simulink model "create_rc_params_Preq"  (Simulink 3.00)
settings: Solver=ode1  StartTime=starttime  StopTime=endtime  FixedStep=0.5  RelTol=1e-3
values from neighbouring files (symbols this model uses):
  cb = energy/(0.5*(Vmax^2-Vmin^2))    [process_HPPC.m]
  cc = tau/(re+rt)    [process_HPPC.m]
  ess_max_volts = template_max_volts    [ESS_RC_template.m]    (also in ESS_template.m)
  ess_min_volts = template_min_volts    [ESS_RC_template.m]    (also in ESS_template.m)
  ess_mod_airflow = max(ess_mod_airflow,0.001)    [ESS_RC_template.m]    (also in ESS_template.m)
  ess_mod_cp = template_mod_cp    [ESS_RC_template.m]    (also in ESS_template.m)
  ess_module_mass = template_module_mass    [ESS_RC_template.m]    (also in ESS_template.m)
  ess_module_num = template_module_num    [ESS_RC_template.m]    (also in ESS_template.m)
  ess_set_tmp = template_set_tmp    [ESS_RC_template.m]    (also in ESS_template.m)
  ess_soc = template_soc    [ESS_RC_template.m]    (also in ESS_template.m; make_ADV_RC_bat_file.m = binf.VOC.ess_soc/100; make_ADV_bat_file.m = binf.VOC.ess_soc; process_HPPC.m = [0:.2:min_soc-.2 min_soc:.05:max_soc max_soc+.2:.2:1])
  ess_th_calc = 1    [ESS_RC_template.m]    (also in ESS_template.m)
  ess_th_res_off = ((1/4)+(ess_mod_case_thk/ess_mod_case_th_cond))/ess_mod_sarea    [ESS_RC_template.m]    (also in ESS_template.m)
  ess_th_res_on = min(ess_th_res_on,ess_th_res_off)    [ESS_RC_template.m]    (also in ESS_template.m)
  ess_tmp = template_tmp    [ESS_RC_template.m]    (also in ESS_template.m; process_HPPC.m = [1 1.01]*Temperature)
  ess_voc = template_voc    [ESS_RC_template.m]    (also in ESS_template.m = template_voc*templatenum_cells_per_mod; process_HPPC.m = [ess_voc_data;ess_voc_data]; process_data.m = binf.VOC.ess_voc)
  mc_min_volts = 0    [validate_rc.m]
  rc = Rbulk/3.732*factor    [process_HPPC.m]
  re = Rbulk/(1.244)    [process_HPPC.m]
  rt = Rbulk/1.368*factor    [process_HPPC.m]
undefined symbols (not defined in the file or in its folder): air_cp, amb_tmp, cyc_mph, ess_init_soc, ess_mod_init_tmp, power_data, time_data
settings Model: LastModifiedBy=vjohnson

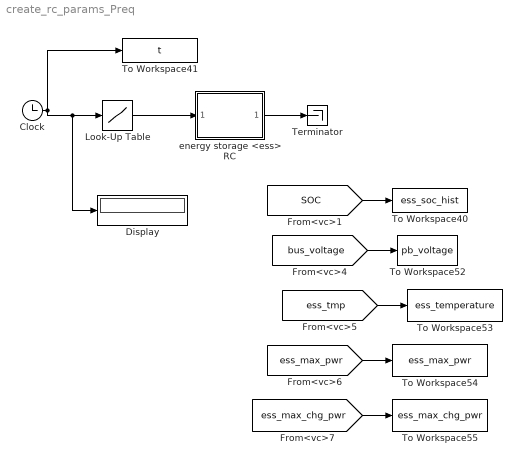
== system create_rc_params_Preq ==
  Clock : Clock
      settings: DisplayTime=off  Decimation=10
  Display : Display
      settings: Format=short
  Look-Up Table : Lookup  InputValues=time_data  OutputValues=power_data
  Terminator : Terminator
  To Workspace40 : ToWorkspace  VariableName=ess_soc_hist  SampleTime=-1  SaveFormat=Matrix
  To Workspace41 : ToWorkspace  VariableName=t  SampleTime=-1  SaveFormat=Matrix
  To Workspace52 : ToWorkspace  VariableName=pb_voltage  SampleTime=-1  SaveFormat=Matrix
  To Workspace53 : ToWorkspace  VariableName=ess_temperature  SampleTime=-1  SaveFormat=Matrix
  To Workspace54 : ToWorkspace  VariableName=ess_max_pwr  SampleTime=-1  SaveFormat=Matrix
  To Workspace55 : ToWorkspace  VariableName=ess_max_chg_pwr  SampleTime=-1  SaveFormat=Matrix
  energy storage <ess> RC : Subsystem
      mask Display: image(imread('bdi_ess.jpg'))
  wires:
  Look-Up Table/1 -> energy storage <ess> RC/1(power req'd into bus (W))
  energy storage <ess> RC/1(power available to bus (W)) -> Terminator/1
  [bus_voltage] -> To Workspace52/1
  [SOC] -> To Workspace40/1
  [ess_tmp] -> To Workspace53/1
  [ess_max_pwr] -> To Workspace54/1
  [ess_max_chg_pwr] -> To Workspace55/1
  Clock/1 -> To Workspace41/1, Look-Up Table/1, Display/1

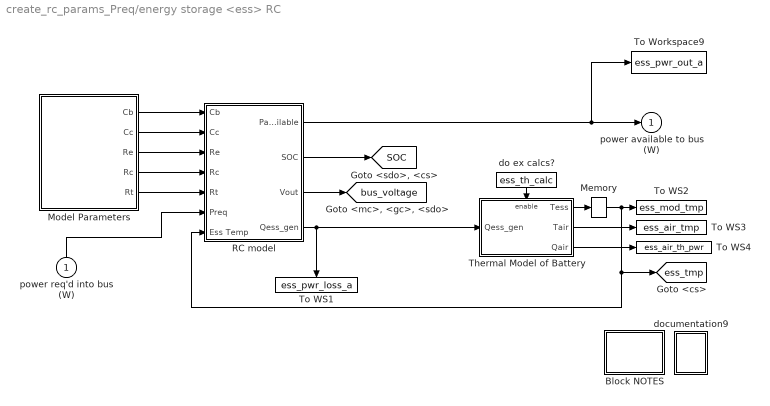
== system create_rc_params_Preq/energy storage <ess> RC ==
  power req'd into bus (W) : Inport  Orientation=up  Port=1  PortWidth=-1  SampleTime=-1  DataType=auto
      settings: SignalType=auto
  Block NOTES : Subsystem
      mask Display: disp('Block\nNOTES')
  Memory : Memory  X0=ess_mod_init_tmp  InheritSampleTime=off
  Model Parameters : Subsystem
  RC model : Subsystem
  Thermal Model of Battery : Subsystem
  To WS1 : ToWorkspace  VariableName=ess_pwr_loss_a  SampleTime=0  SaveFormat=Matrix
      settings: Orientation=down
  To WS2 : ToWorkspace  VariableName=ess_mod_tmp  SampleTime=0  SaveFormat=Matrix
  To WS3 : ToWorkspace  VariableName=ess_air_tmp  SampleTime=0  SaveFormat=Matrix
  To WS4 : ToWorkspace  VariableName=ess_air_th_pwr  SampleTime=0  SaveFormat=Matrix
  To Workspace9 : ToWorkspace  VariableName=ess_pwr_out_a  SampleTime=-1  SaveFormat=Matrix
  do ex calcs? : Constant  Orientation=down  Value=ess_th_calc
  documentation9 : Subsystem
      settings: OpenFcn=web(['file:\\\' which('energy_storage.htm')]);
      mask Display: image(imread('doc_man.jpg'))
  power available to bus (W) : Outport  Port=1  InitialOutput=0
  tag scope: SOC=global, bus_voltage=global, ess_tmp=global
  wires:
  Model Parameters/1(Cb) -> RC model/1(Cb)
  Model Parameters/2(Cc) -> RC model/2(Cc)
  Model Parameters/3(Re) -> RC model/3(Re)
  Model Parameters/4(Rc) -> RC model/4(Rc)
  Model Parameters/5(Rt) -> RC model/5(Rt)
  RC model/3(Vout) -> [bus_voltage]
  RC model/4(Qess_gen) -> To WS1/1, Thermal Model of Battery/1(Qess_gen)
  Memory/1 -> To WS2/1, [ess_tmp], RC model/7(Ess Temp)
  Thermal Model of Battery/1(Tess) -> Memory/1
  Thermal Model of Battery/3(Qair) -> To WS4/1
  Thermal Model of Battery/2(Tair) -> To WS3/1
  do ex calcs?/1 -> Thermal Model of Battery/Enable
  RC model/1(Pavailable) -> power available to bus (W)/1, To Workspace9/1
  power req'd into bus (W)/1 -> RC model/6(Preq)
  RC model/2(SOC) -> [SOC]

== system create_rc_params_Preq/energy storage <ess> RC/Block NOTES ==
  note: This block models the energy storage system as an SOC-dependent voltage
      | in series with an SOC- and current direction-dependent internal resistance.
      | SOC is computed assuming that A-h capacity is constant, but limited
      | such that a minimum voltage is never exceeded (replacing the
      | previous Peukert relationship which underpredicted battery capacity).
      |
      | Discharge power is limited here so as not to bring the bus (battery pack) voltage below
      | the minimum controller voltage or the minimum battery voltage and so as to allow
      | the solution of the quadratic eq'n for discharge current.
      |
      | Charge current is limited to ensure the voltage does not exceed a maximum
      | voltage
      |
      | Positive current is discharge current in the convention used here.
      | Power loss is computed as I*R+losses due to Coulombic (in)efficiency.
      |
      | Thermal modeling of the battery performance is modeled in the
      | OCV, Rint, and capacity.

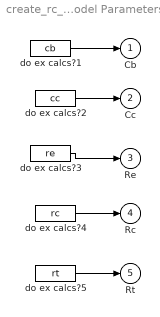
== system create_rc_params_Preq/energy storage <ess> RC/Model Parameters ==
  do ex calcs?1 : Constant  Value=cb
  do ex calcs?2 : Constant  Value=cc
  do ex calcs?3 : Constant  Value=re
  do ex calcs?4 : Constant  Value=rc
  do ex calcs?5 : Constant  Value=rt
  Cb : Outport  Port=1  InitialOutput=0
  Cc : Outport  Port=2  InitialOutput=0
  Re : Outport  Port=3  InitialOutput=0
  Rc : Outport  Port=4  InitialOutput=0
  Rt : Outport  Port=5  InitialOutput=0
  wires:
  do ex calcs?1/1 -> Cb/1
  do ex calcs?2/1 -> Cc/1
  do ex calcs?3/1 -> Re/1
  do ex calcs?5/1 -> Rt/1
  do ex calcs?4/1 -> Rc/1

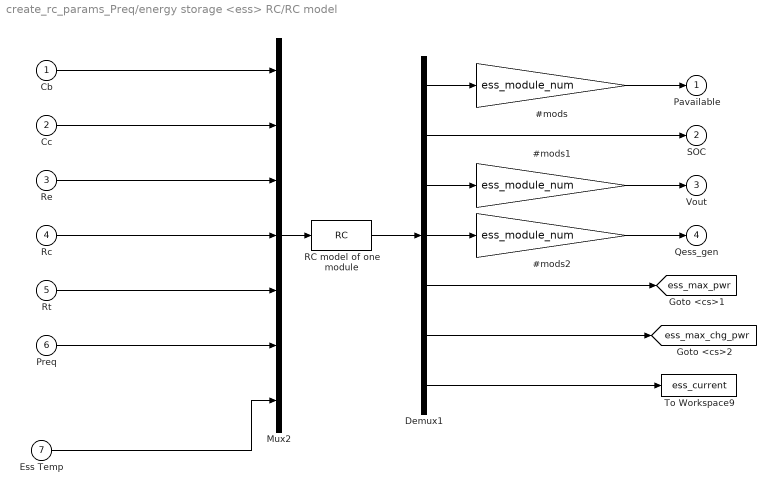
== system create_rc_params_Preq/energy storage <ess> RC/RC model ==
  Cb : Inport  Port=1  PortWidth=-1  SampleTime=-1  DataType=auto
      settings: SignalType=auto
  Cc : Inport  Port=2  PortWidth=-1  SampleTime=-1  DataType=auto
      settings: SignalType=auto
  Re : Inport  Port=3  PortWidth=-1  SampleTime=-1  DataType=auto
      settings: SignalType=auto
  Rc : Inport  Port=4  PortWidth=-1  SampleTime=-1  DataType=auto
      settings: SignalType=auto
  Rt : Inport  Port=5  PortWidth=-1  SampleTime=-1  DataType=auto
      settings: SignalType=auto
  Preq : Inport  Port=6  PortWidth=-1  SampleTime=-1  DataType=auto
      settings: SignalType=auto
  Ess Temp : Inport  Port=7  PortWidth=-1  SampleTime=-1  DataType=auto
      settings: SignalType=auto
  #mods : Gain  Gain=ess_module_num  SaturateOnIntegerOverflow=on
  #mods1 : Gain  Gain=ess_module_num  SaturateOnIntegerOverflow=on
  #mods2 : Gain  Gain=ess_module_num  SaturateOnIntegerOverflow=on
  Demux1 : Demux  Outputs=7
  Mux2 : Mux  Inputs=7
      settings: DisplayOption=none
  RC model of one module : S-Function  FunctionName=RC  Parameters=ess_min_volts,ess_max_volts,mc_min_volts,ess_soc,ess_tmp,ess_voc,ess_init_soc,ess_mod_init_tmp  PortCounts=[]  SFunctionModules=''
  To Workspace9 : ToWorkspace  VariableName=ess_current  SampleTime=-1  SaveFormat=Matrix
  Pavailable : Outport  Port=1  InitialOutput=0
  SOC : Outport  Port=2  InitialOutput=0
  Vout : Outport  Port=3  InitialOutput=0
  Qess_gen : Outport  Port=4  InitialOutput=0
  tag scope: ess_max_chg_pwr=global, ess_max_pwr=global
  wires:
  Cb/1 -> Mux2/1
  Cc/1 -> Mux2/2
  Re/1 -> Mux2/3
  Rc/1 -> Mux2/4
  Rt/1 -> Mux2/5
  Mux2/1 -> RC model of one module/1
  Demux1/2 -> SOC/1
  Demux1/1 -> #mods/1
  #mods/1 -> Pavailable/1
  Demux1/3 -> #mods1/1
  #mods1/1 -> Vout/1
  Demux1/4 -> #mods2/1
  #mods2/1 -> Qess_gen/1
  Demux1/5 -> [ess_max_pwr]
  Demux1/6 -> [ess_max_chg_pwr]
  RC model of one module/1 -> Demux1/1
  Preq/1 -> Mux2/6
  Demux1/7 -> To Workspace9/1
  Ess Temp/1 -> Mux2/7

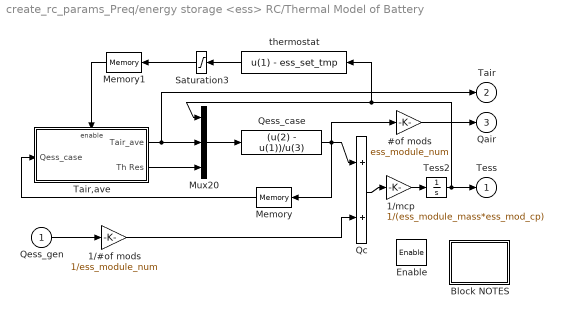
== system create_rc_params_Preq/energy storage <ess> RC/Thermal Model of Battery ==
  Qess_gen : Inport  Port=1  PortWidth=-1  SampleTime=-1  DataType=auto
      settings: SignalType=auto
  Enable : EnablePort  StatesWhenEnabling=reset
  #of mods : Gain  Gain=ess_module_num  SaturateOnIntegerOverflow=on
  1/#of mods : Gain  Gain=1/ess_module_num  SaturateOnIntegerOverflow=on
  1/mcp : Gain  Gain=1/(ess_module_mass*ess_mod_cp)  SaturateOnIntegerOverflow=on
  Block NOTES : Subsystem
      mask Display: disp('Block\nNOTES')
  Memory : Memory  Orientation=left  X0=cyc_mph(1,2)*.447  InheritSampleTime=off
  Memory1 : Memory  Orientation=left  X0=cyc_mph(1,2)*.447  InheritSampleTime=off
  Mux20 : Mux  Inputs=3
      settings: DisplayOption=none
  Qc : Sum  Inputs=++  SaturateOnIntegerOverflow=on
  Qess_case : Fcn  Expr=(u(2) - u(1))/u(3)
  Saturation3 : Saturate  Orientation=left  UpperLimit=1  LowerLimit=0
  Tair,ave : Subsystem
  Tess2 : Integrator  ExternalReset=none  InitialConditionSource=internal  InitialCondition=ess_mod_init_tmp  LimitOutput=off  UpperSaturationLimit=inf  LowerSaturationLimit=-inf  ShowSaturationPort=off  ShowStatePort=off  AbsoluteTolerance=auto
  thermostat : Fcn  Orientation=left  Expr=u(1) - ess_set_tmp
  Tess : Outport  Port=1  InitialOutput=0
  Tair : Outport  Port=2
  Qair : Outport  Port=3  OutputWhenDisabled=reset  InitialOutput=0
  wires:
  Qc/1 -> 1/mcp/1
  Qess_case/1 -> Qc/1, Memory/1, #of mods/1
  1/mcp/1 -> Tess2/1
  Tess2/1 -> Tess/1, Mux20/1, thermostat/1
  Qess_gen/1 -> 1/#of mods/1
  1/#of mods/1 -> Qc/2
  thermostat/1 -> Saturation3/1
  Saturation3/1 -> Memory1/1
  Memory1/1 -> Tair,ave/Enable
  Memory/1 -> Tair,ave/1(Qess_case)
  #of mods/1 -> Qair/1
  Mux20/1 -> Qess_case/1
  Tair,ave/2(Th Res) -> Mux20/3
  Tair,ave/1(Tair_ave) -> Mux20/2, Tair/1

== system create_rc_params_Preq/energy storage <ess> RC/documentation9 ==

== system create_rc_params_Preq/energy storage <ess> RC/Thermal Model of Battery/Block NOTES ==
  note: This block models the thermal behavior of a battery module with active air cooling.
      | The module is modeled as a single lumped thermal mass.
      | The fan is on whenever the battery temp is > the set temp.

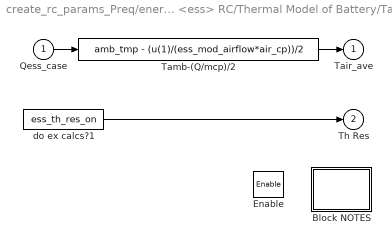
== system create_rc_params_Preq/energy storage <ess> RC/Thermal Model of Battery/Tair,ave ==
  Qess_case : Inport  Port=1  PortWidth=-1  SampleTime=-1  DataType=auto
      settings: SignalType=auto
  Enable : EnablePort  StatesWhenEnabling=reset
  Block NOTES : Subsystem
      mask Display: disp('Block\nNOTES')
  Tamb-(Q/mcp)/2 : Fcn  Expr=amb_tmp - (u(1)/(ess_mod_airflow*air_cp))/2
  do ex calcs?1 : Constant  Value=ess_th_res_on
  Tair_ave : Outport  Port=1  OutputWhenDisabled=reset  InitialOutput=amb_tmp
  Th Res : Outport  Port=2  OutputWhenDisabled=reset  InitialOutput=ess_th_res_off
  wires:
  Tamb-(Q/mcp)/2/1 -> Tair_ave/1
  Qess_case/1 -> Tamb-(Q/mcp)/2/1
  do ex calcs?1/1 -> Th Res/1

== system create_rc_params_Preq/energy storage <ess> RC/Thermal Model of Battery/Tair,ave/Block NOTES ==
  note: This block determins the average temperature of the cooling air over the module.
